simulink model "effect_zeta_dampingratio"  (R2023b)
settings: Solver=VariableStepAuto  StartTime=0.0  StopTime=10.0  RelTol=1e-3
settings Model: Creator=hp  LastModifiedBy=hp

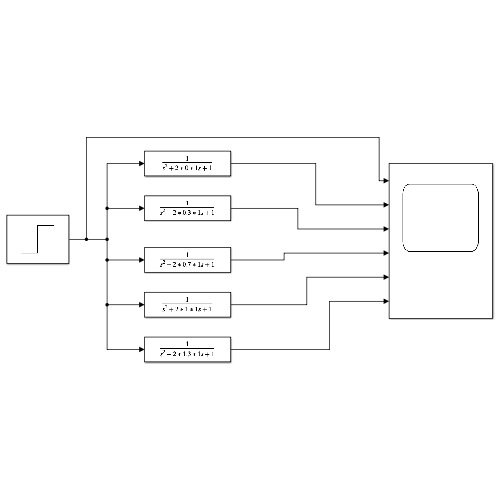
[thumbnail: Simulink's stored preview of the top-level diagram]
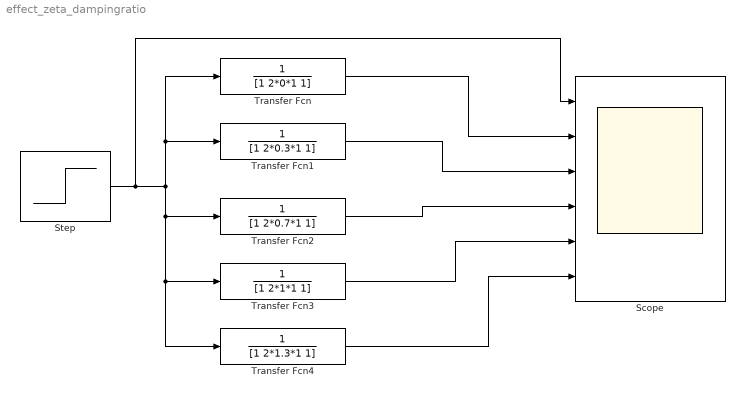
== system effect_zeta_dampingratio ==
  Scope : Scope  NumInputPorts=6
  Step : Step  SampleTime=0
  Transfer Fcn : TransferFcn  Denominator=[1 2*0*1 1]
  Transfer Fcn1 : TransferFcn  Denominator=[1 2*0.3*1 1]
  Transfer Fcn2 : TransferFcn  Denominator=[1 2*0.7*1 1]
  Transfer Fcn3 : TransferFcn  Denominator=[1 2*1*1 1]
  Transfer Fcn4 : TransferFcn  Denominator=[1 2*1.3*1 1]
  wires:
  Step/1 -> Scope/1, Transfer Fcn4/1, Transfer Fcn3/1, Transfer Fcn2/1, Transfer Fcn1/1, Transfer Fcn/1
  Transfer Fcn/1 -> Scope/2
  Transfer Fcn1/1 -> Scope/3
  Transfer Fcn2/1 -> Scope/4
  Transfer Fcn3/1 -> Scope/5
  Transfer Fcn4/1 -> Scope/6
